simulink model "LQR_SIP_simulation"  (R2024b)
settings: Solver=ode4  StartTime=0.0  StopTime=10  FixedStep=0.002  RelTol=1e-3  AbsTol=1e-6  EnableMultiTasking=on
undefined symbols (not defined in the file): A, B, C, D, K, wcf, zetaf
libraries: simulink_extras x2
settings Model: ExtModeTrigDuration=5000  Creator=MLevis  LastModifiedBy=Thoma
settings SolverCC: AutoScaleAbsTol=off  AlgebraicLoopSolver=TrustRegion  PositivePriorityOrder=on
settings DataIOCC: SaveFormat=Array  SignalLoggingSaveFormat=ModelDataLogs  ReturnWorkspaceOutputs=off
settings OptimizationCC: BooleanDataType=off  OptimizeBlockIOStorage=off  BufferReuse=off  ExpressionFolding=off  ExpressionDepthLimit=2147483647  LocalBlockOutputs=off  InitFltsAndDblsToZero=on  LifeSpan=inf
settings DebuggingCC: SaveWithParameterizedLinksMsg=none  UnderspecifiedInitializationDetection=Classic  MergeDetectMultiDrivingBlocksExec=none  SignalResolutionControl=TryResolveAllWithWarning  MultiTaskDSMMsg=warning  MultiTaskCondExecSysMsg=none  FcnCallInpInsideContextMsg=warning  UnconnectedInputMsg=warning  UnconnectedOutputMsg=warning  UnconnectedLineMsg=warning  StateNameClashWarn=warning  SFUnexpectedBacktrackingDiag=warning  SFNoUnconditionalDefaultTransitionDiag=warning  SFExecutionAtInitializationDiag=none  ArithmeticOperatorsInVariantConditions=warning
settings HardwareCC: ProdBitPerPointer=32  ProdBitPerSizeT=32  ProdBitPerPtrDiffT=32  ProdLargestAtomicFloat=None  ProdIntDivRoundTo=Undefined  ProdEndianess=Unspecified  ProdWordSize=32  ProdHWDeviceType=32-bit Generic
settings ModelReferenceCC: PropagateSignalLabelsOutOfModel=off
settings SFSimCC: SimUseLocalCustomCode=off  CustomCodeUndefinedFunction=UseInterfaceOnly
settings RTWCC: Description=QUARC Win32 Target  SystemTargetFile=quarc_windows.tlc  TemplateMakefile=quarc_default_tmf  RTWUseLocalCustomCode=off  GPUComputeCapability=3.5
settings CodeAppCC: StateflowObjectComments=on
settings STFCustomTargetCC: TargetFcnLib=ansi_tfl_tmw.mat  TargetPreCompLibLocation=C:\PROGRA~2\QUARC\lib\2011b\windows\release  CPPClassGenCompliant=on  GRTInterface=on  SystemTargetFile=quarc_windows.tlc
settings GRTTargetCC: TargetFcnLib=ansi_tfl_tmw.mat  TargetPreCompLibLocation=C:\PROGRA~2\QUARC\lib\2011b\windows\release  TargetLangStandard=C89/C90 (ANSI)  ParMdlRefBuildCompliant=off  CompOptLevelCompliant=off  ConcurrentExecutionCompliant=off  CombineOutputUpdateFcns=off  MatFileLogging=off  GRTInterface=on  UseToolchainInfoCompliant=off  ExtMode=on  ExtModeMexFile=quarc_comm
settings ConfigComp: CovMetricSettings=dw  CovSaveCumulativeToWorkspaceVar=on  CovSaveSingleToWorkspaceVar=on  CovExternalEMLEnable=off

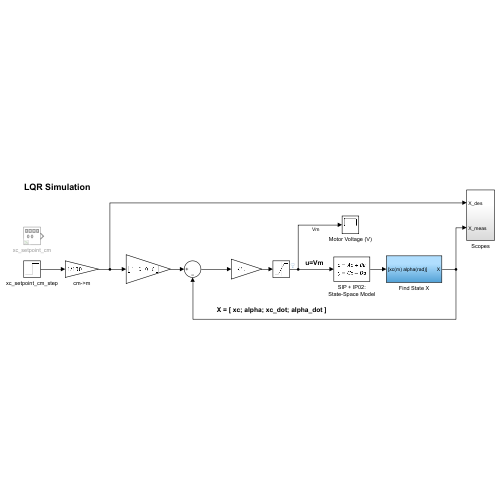
[thumbnail: Simulink's stored preview of the top-level diagram]
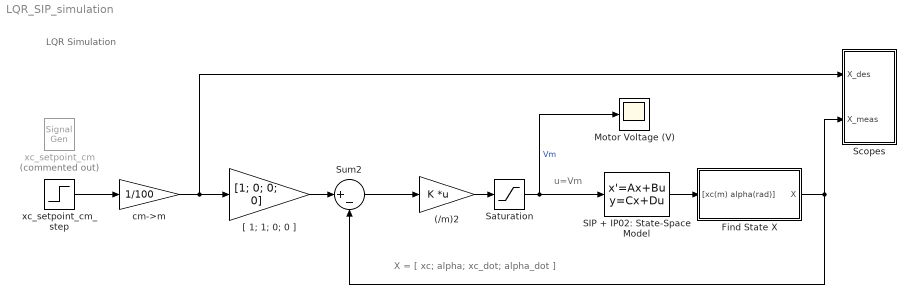
== system LQR_SIP_simulation ==
  note: LQR Simulation
  note: u=Vm
  note: X = [ xc; alpha; xc_dot; alpha_dot ]
  (/m)2 : Gain  Gain=K  Multiplication=Matrix(K*u)  SaturateOnIntegerOverflow=on  OutDataTypeStr=Inherit: Same as input  ParamDataTypeStr=Inherit: Same as input
  Find State X : Subsystem
  Motor Voltage (V) : Scope
  SIP + IP02: State-Space Model : StateSpace  A=A  B=B  C=C  D=D  InitialCondition=[-0.0162197; deg2rad(-0.175718); -0.0277821; deg2rad(-0.569332)]
  Saturation : Saturate  UpperLimit=10  LowerLimit=-10
  Scopes : Subsystem
  Sum2 : Sum  Inputs=|+-  InputSameDT=on  SaturateOnIntegerOverflow=on  OutDataTypeStr=Inherit: Same as first input
  "[ 1; 1; 0; 0 ]" : Gain  Gain=[1; 0; 0; 0]  SaturateOnIntegerOverflow=on  OutDataTypeStr=Inherit: Same as input  ParamDataTypeStr=Inherit: Same as input
  cm->m : Gain  Gain=1/100
  xc_setpoint_cm : SignalGenerator  Commented=on  Amplitude=10  Frequency=0.1
  xc_setpoint_cm_step : Step  Time=0  After=20  SampleTime=0
  wires:
  (/m)2/1 -> Saturation/1
  Sum2/1 -> (/m)2/1
  Saturation/1 -> SIP + IP02: State-Space Model/1, Motor Voltage (V)/1  "Vm"
  SIP + IP02: State-Space Model/1 -> Find State X/1("[xc(m) alpha(rad)]")
  Find State X/1(X) -> Scopes/2(X_meas), Sum2/2
  "[ 1; 1; 0; 0 ]"/1 -> Sum2/1
  cm->m/1 -> Scopes/1(X_des), "[ 1; 1; 0; 0 ]"/1
  xc_setpoint_cm_step/1 -> cm->m/1

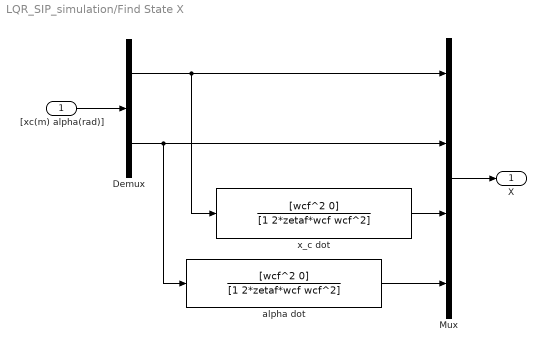
== system LQR_SIP_simulation/Find State X ==
  "[xc(m) alpha(rad)]" : Inport
  Demux : Demux  Outputs=2
  Mux : Mux
  alpha dot : TransferFcn  Numerator=[wcf^2 0]  Denominator=[1 2*zetaf*wcf wcf^2]
  x_c dot : TransferFcn  Numerator=[wcf^2 0]  Denominator=[1 2*zetaf*wcf wcf^2]
  X : Outport
  wires:
  Mux/1 -> X/1
  x_c dot/1 -> Mux/3
  alpha dot/1 -> Mux/4
  "[xc(m) alpha(rad)]"/1 -> Demux/1
  Demux/1 -> x_c dot/1, Mux/1
  Demux/2 -> Mux/2, alpha dot/1

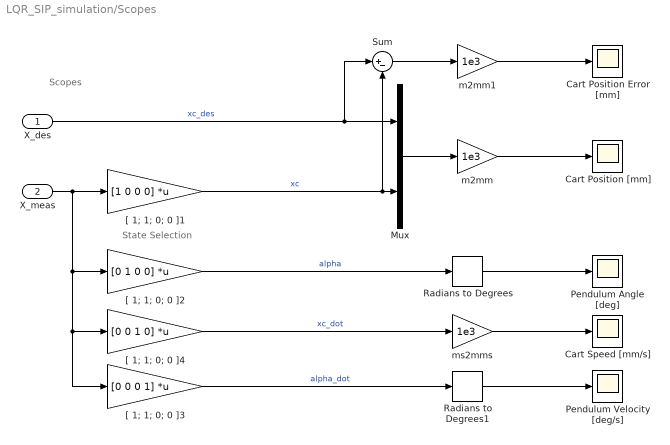
== system LQR_SIP_simulation/Scopes ==
  note: State Selection
  note: Scopes
  X_des : Inport
  X_meas : Inport  Port=2
  Cart Position Error [mm] : Scope
  Cart Position [mm] : Scope
  Cart Speed [mm/s] : Scope
  Mux : Mux  Inputs=2
  Pendulum Angle [deg] : Scope
  Pendulum Velocity [deg/s] : Scope
  Radians to Degrees : simulink_extras/Transformations/Radians to Degrees
  Radians to Degrees1 : simulink_extras/Transformations/Radians to Degrees
  Sum : Sum  Inputs=|+-
  "[ 1; 1; 0; 0 ]1" : Gain  Gain=[1 0 0 0]  Multiplication=Matrix(K*u)  SaturateOnIntegerOverflow=on  OutDataTypeStr=Inherit: Same as input  ParamDataTypeStr=Inherit: Same as input
  "[ 1; 1; 0; 0 ]2" : Gain  Gain=[0 1 0 0]  Multiplication=Matrix(K*u)  SaturateOnIntegerOverflow=on  OutDataTypeStr=Inherit: Same as input  ParamDataTypeStr=Inherit: Same as input
  "[ 1; 1; 0; 0 ]3" : Gain  Gain=[0 0 0 1]  Multiplication=Matrix(K*u)  SaturateOnIntegerOverflow=on  OutDataTypeStr=Inherit: Same as input  ParamDataTypeStr=Inherit: Same as input
  "[ 1; 1; 0; 0 ]4" : Gain  Gain=[0 0 1 0]  Multiplication=Matrix(K*u)  SaturateOnIntegerOverflow=on  OutDataTypeStr=Inherit: Same as input  ParamDataTypeStr=Inherit: Same as input
  m2mm : Gain  Gain=1e3  SaturateOnIntegerOverflow=on  OutDataTypeStr=Inherit: Same as input  ParamDataTypeStr=Inherit: Same as input
  m2mm1 : Gain  Gain=1e3  SaturateOnIntegerOverflow=on  OutDataTypeStr=Inherit: Same as input  ParamDataTypeStr=Inherit: Same as input
  ms2mms : Gain  Gain=1e3  SaturateOnIntegerOverflow=on  OutDataTypeStr=Inherit: Same as input  ParamDataTypeStr=Inherit: Same as input
  wires:
  Mux/1 -> m2mm/1
  m2mm/1 -> Cart Position [mm]/1
  "[ 1; 1; 0; 0 ]1"/1 -> Sum/2, Mux/2  "xc"
  X_meas/1 -> "[ 1; 1; 0; 0 ]1"/1, "[ 1; 1; 0; 0 ]3"/1, "[ 1; 1; 0; 0 ]4"/1, "[ 1; 1; 0; 0 ]2"/1
  Radians to Degrees/1 -> Pendulum Angle [deg]/1
  X_des/1 -> Sum/1, Mux/1  "xc_des"
  "[ 1; 1; 0; 0 ]2"/1 -> Radians to Degrees/1  "alpha"
  m2mm1/1 -> Cart Position Error [mm]/1
  Sum/1 -> m2mm1/1
  "[ 1; 1; 0; 0 ]3"/1 -> Radians to Degrees1/1  "alpha_dot"
  Radians to Degrees1/1 -> Pendulum Velocity [deg/s]/1
  ms2mms/1 -> Cart Speed [mm/s]/1
  "[ 1; 1; 0; 0 ]4"/1 -> ms2mms/1  "xc_dot"
